simulink model "IMU_Sim"  (R2021a)
settings: Solver=FixedStepAuto  StartTime=0.0  StopTime=6000.0  FixedStep=0.1  RelTol=1e-3
libraries: mspsensorlib x1
settings Model: Creator=panch  LastModifiedBy=panch

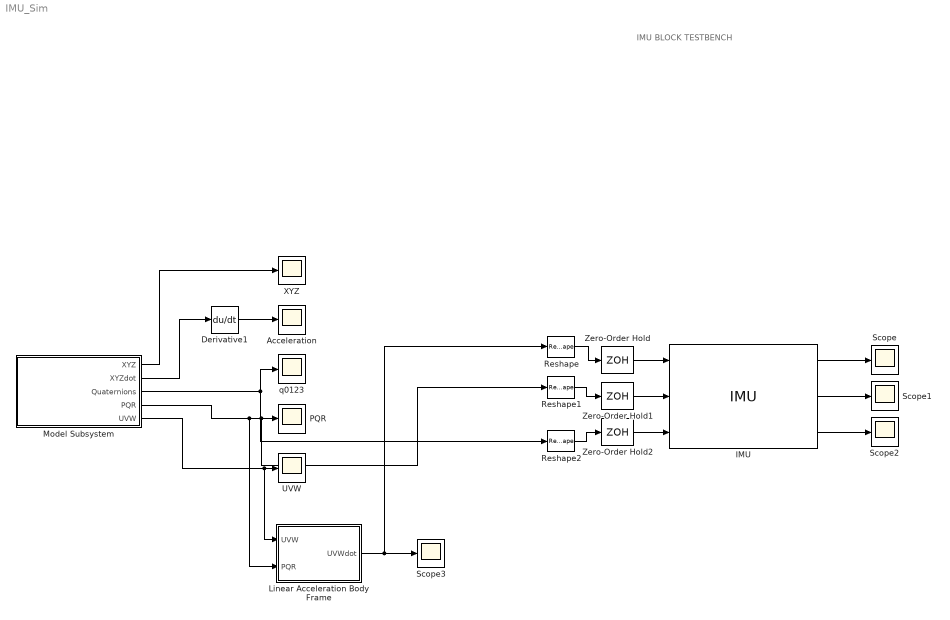
== system IMU_Sim ==
  note: IMU BLOCK TESTBENCH
  Acceleration : Scope
  Derivative1 : Derivative
  IMU : mspsensorlib/IMU  DispRefFrame=NED  Temperature=0  MagneticFieldNED=[27.5550, -2.4169, -16.0849]  MagneticFieldENU=[ -2.4169, 27.5550, 16.0849 ]  SeedDouble=67  SimulateUsing=Code generation  AccelParamsMeasurementRange=Inf  AccelParamsResolution=0  AccelParamsConstantBias=[ 0, 0, 0 ]  AccelParamsAxesMisalignment=[ 0, 0, 0 ]  AccelParamsNoiseDensity=[ 0, 0, 0 ]  AccelParamsBiasInstability=[ 0, 0, 0 ]  AccelParamsRandomWalk=[ 0, 0, 0 ]  AccelParamsTemperatureBias=[ 0, 0, 0 ]  AccelParamsTemperatureScaleFactor=[ 0, 0, 0 ]  GyroParamsMeasurementRange=Inf  GyroParamsResolution=0  GyroParamsConstantBias=[ 0, 0, 0 ]  GyroParamsAxesMisalignment=[ 0, 0, 0 ]  GyroParamsAccelerationBias=[ 0, 0, 0 ]  GyroParamsNoiseDensity=[ 0, 0, 0 ]  GyroParamsBiasInstability=[ 0, 0, 0 ]  GyroParamsRandomWalk=[ 0, 0, 0 ]  GyroParamsTemperatureBias=[ 0, 0, 0 ]  GyroParamsTemperatureScaleFactor=[ 0, 0, 0 ]  MagParamsMeasurementRange=Inf  MagParamsResolution=0  MagParamsConstantBias=[ 0, 0, 0 ]  MagParamsAxesMisalignment=[ 0, 0, 0 ]  MagParamsNoiseDensity=[ 0, 0, 0 ]  MagParamsBiasInstability=[ 0, 0, 0 ]  MagParamsRandomWalk=[ 0, 0, 0 ]  MagParamsTemperatureBias=[ 0, 0, 0 ]  MagParamsTemperatureScaleFactor=[ 0, 0, 0 ]
      settings: SourceProductBaseCode=TF,NV
  Linear Acceleration Body Frame : Subsystem
  Model Subsystem : Subsystem
  PQR : Scope
  Reshape : Reshape  OutputDimensionality=Customize  OutputDimensions=[1,3]
  Reshape1 : Reshape  OutputDimensionality=Customize  OutputDimensions=[1,3]
  Reshape2 : Reshape  OutputDimensionality=Customize  OutputDimensions=[1,4]
  Scope{,1..3} (4 alike) : Scope
  UVW : Scope
  XYZ : Scope
  Zero-Order Hold : ZeroOrderHold  SampleTime=-1
  Zero-Order Hold1 : ZeroOrderHold  SampleTime=-1
  Zero-Order Hold2 : ZeroOrderHold  SampleTime=-1
  q0123 : Scope
  wires:
  Reshape/1 -> Zero-Order Hold/1
  Zero-Order Hold/1 -> IMU/1
  Reshape1/1 -> Zero-Order Hold1/1
  Reshape2/1 -> Zero-Order Hold2/1
  Zero-Order Hold2/1 -> IMU/3
  IMU/1 -> Scope/1
  IMU/2 -> Scope1/1
  IMU/3 -> Scope2/1
  Zero-Order Hold1/1 -> IMU/2
  Model Subsystem/1(XYZ) -> XYZ/1
  Model Subsystem/2(XYZdot) -> Derivative1/1
  Derivative1/1 -> Acceleration/1
  Model Subsystem/3(Quaternions) -> q0123/1, Reshape2/1
  Model Subsystem/4(PQR) -> Reshape1/1, PQR/1, Linear Acceleration Body Frame/2(PQR)
  Model Subsystem/5(UVW) -> Linear Acceleration Body Frame/1(UVW), UVW/1
  Linear Acceleration Body Frame/1(UVWdot) -> Reshape/1, Scope3/1

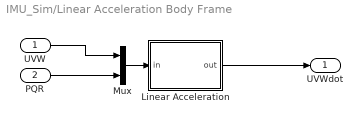
== system IMU_Sim/Linear Acceleration Body Frame ==
  UVW : Inport
  PQR : Inport  Port=2
  Linear Acceleration : MATLAB Function  TreatAsAtomicUnit=on
  Mux : Mux  Inputs=2
  UVWdot : Outport
  wires:
  Mux/1 -> Linear Acceleration/1(in)
  Linear Acceleration/1(out) -> UVWdot/1
  UVW/1 -> Mux/1
  PQR/1 -> Mux/2

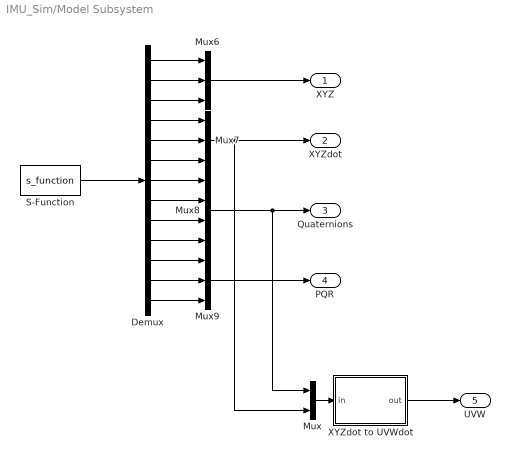
== system IMU_Sim/Model Subsystem ==
  Demux : Demux  Outputs=13
  Mux : Mux  Inputs=2
  Mux6 : Mux  Inputs=3
  Mux7 : Mux  Inputs=3
  Mux8 : Mux
  Mux9 : Mux  Inputs=3
  S-Function : S-Function  FunctionName=s_function  SFunctionDeploymentMode=off  EnableBusSupport=off
  XYZdot to UVWdot : MATLAB Function  TreatAsAtomicUnit=on
  XYZ : Outport
  XYZdot : Outport  Port=2
  Quaternions : Outport  Port=3
  PQR : Outport  Port=4
  UVW : Outport  Port=5
  wires:
  S-Function/1 -> Demux/1
  Demux/8 -> Mux8/2
  Demux/4 -> Mux7/1
  Demux/11 -> Mux9/1
  Demux/10 -> Mux8/4
  Demux/1 -> Mux6/1
  Demux/5 -> Mux7/2
  Demux/2 -> Mux6/2
  Demux/9 -> Mux8/3
  Demux/12 -> Mux9/2
  Demux/13 -> Mux9/3
  Mux6/1 -> XYZ/1
  Demux/7 -> Mux8/1
  Demux/3 -> Mux6/3
  Demux/6 -> Mux7/3
  Mux9/1 -> PQR/1
  Mux7/1 -> Mux/2, XYZdot/1
  Mux8/1 -> Mux/1, Quaternions/1
  Mux/1 -> XYZdot to UVWdot/1(in)
  XYZdot to UVWdot/1(out) -> UVW/1

== matlab function IMU_Sim/Model Subsystem/XYZdot to UVWdot ==
  data: in input; out output
function out = fcn(in)

q0 = in(1);
q1 = in(2);
q2 = in(3);
q3 = in(4);
xdot = in(5);
ydot = in(6);
zdot = in(7);

T_mat = TIBquat([q0;q1;q2;q3]).'; % Transponse as we need UVW
out = T_mat * [xdot;ydot;zdot];

== matlab function IMU_Sim/Linear Acceleration Body Frame/Linear Acceleration ==
  data: in input; out output
function out = fcn(in)

u = in(1);
v = in(2);
w = in(3);
p = in(4);
q = in(5);
r = in(6);

% Lookl at Eq 54, we need linear acceleration so without gravity
% XYZ = 0
m = 2.6; %%mass in kilograms
pqr_mat = [0,-r,q;...
           r,0,-p;...
           -q,p,0];
XYZ = [0;0;0];
out = 1/m * XYZ - pqr_mat*[u;v;w];
